simulink model "cell1"  (Simulink 8.1)
settings: Solver=ode45  StartTime=0.0  StopTime=10.0  RelTol=1e-3
values from neighbouring files (symbols this model uses):
  alfa = Cin/(Co+(Co+Cin)/A)    (= 0.999800039992)    [tb1.m]
  gamma = 1/(1+Cin/((A+1)*Co))    (= 0.999900019996)    [tb1.m]
  GBW = 1    [tb1.m]
  SR = 10    [tb1.m]
  Ts = 1    [tb1.m]
  VinHi = 2    [tb1.m]
undefined symbols (not defined in the file or in its folder): slew
settings Model: Creator=yasuda  LastModifiedBy=anagix
settings OptimizationCC: InitFltsAndDblsToZero=on
settings DebuggingCC: SaveWithParameterizedLinksMsg=none  StrictBusMsg=Warning
settings GRTTargetCC: TargetFcnLib=ansi_tfl_tmw.mat

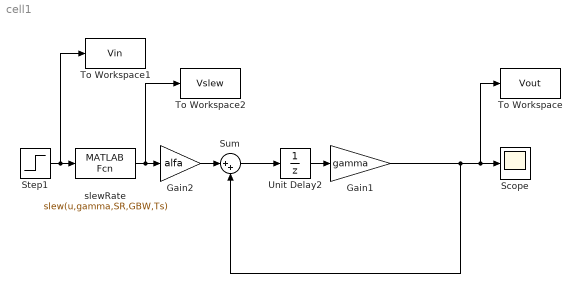
== system cell1 ==
  Gain1 : Gain  Gain=gamma
  Gain2 : Gain  Gain=alfa
  Scope : Scope
  Step1 : Step  After=VinHi  SampleTime=0
  Sum : Sum  Inputs=|++
  To Workspace : ToWorkspace  VariableName=Vout  SampleTime=1
  To Workspace1 : ToWorkspace  VariableName=Vin  SampleTime=1
  To Workspace2 : ToWorkspace  VariableName=Vslew  SampleTime=1
  Unit Delay2 : UnitDelay  SampleTime=Ts
  slewRate : MATLABFcn  MATLABFcn=slew(u,gamma,SR,GBW,Ts)
  wires:
  Sum/1 -> Unit Delay2/1
  Unit Delay2/1 -> Gain1/1
  Gain1/1 -> Sum/2, Scope/1, To Workspace/1
  Gain2/1 -> Sum/1
  slewRate/1 -> Gain2/1, To Workspace2/1
  Step1/1 -> slewRate/1, To Workspace1/1
